simulink model "opencn"  (R2019b)
settings: Solver=FixedStepDiscrete  StartTime=0.0  StopTime=10000  RelTol=1e-3
libraries: libopencn x3, simulink x1
settings Model: PauseTimes=0  Creator=peter  LastModifiedBy=peter
settings HardwareCC: ProdBitPerLong=64  ProdHWDeviceType=Intel->x86-64 (Linux 64)

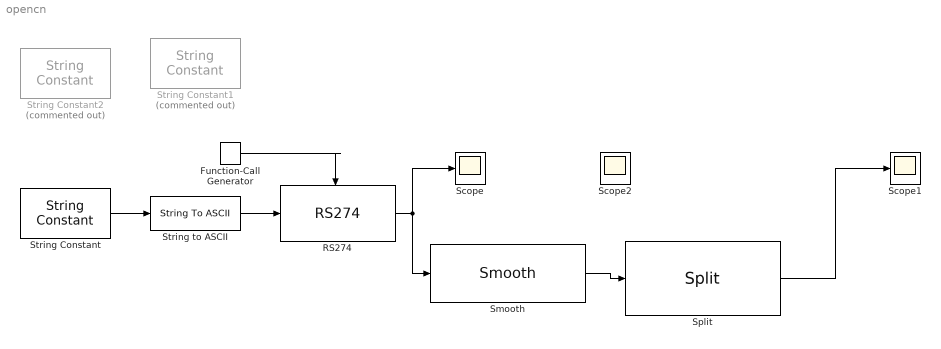
== system opencn ==
  Function-Call Generator : simulink/Ports & Subsystems/Function-Call Generator  sample_time=1  numberOfIterations=1
  "RS274 " : libopencn/RS274   SystemSampleTime=-1  Latency=0  AutoFrameSizeCalculation=off
  Scope : Scope
  Scope1 : Scope
  Smooth : libopencn/Smooth  SystemSampleTime=-1  Latency=0  AutoFrameSizeCalculation=off
  Split : libopencn/Split  SystemSampleTime=-1  Latency=0  AutoFrameSizeCalculation=off
  String Constant : StringConstant  String="\"ngc_test/test_long.ngc\""
  String Constant1 : StringConstant  Commented=on  String="\"ngc_test/PieceDemoLinuxCNC_HV_V05.ngc\""
  String Constant2 : StringConstant  Commented=on  String="\"ngc_test/anchor.ngc\""
  String to ASCII : StringToASCII  OutputVectorSize=255
  Scope2 : Scope
  wires:
  "RS274 "/1 -> Smooth/1, Scope/1
  String Constant/1 -> String to ASCII/1
  Smooth/1 -> Split/1
  String to ASCII/1 -> "RS274 "/1
  Function-Call Generator/1 -> "RS274 "/Trigger
  Split/1 -> Scope1/1
